simulink model "extforce_free_orbit_box"  (R2019b)
settings: Solver=ode45  StartTime=0.0  StopTime=20000.0  MaxStep=0.01  RelTol=1e-8
settings Model: Creator=Hector  LastModifiedBy=Hector

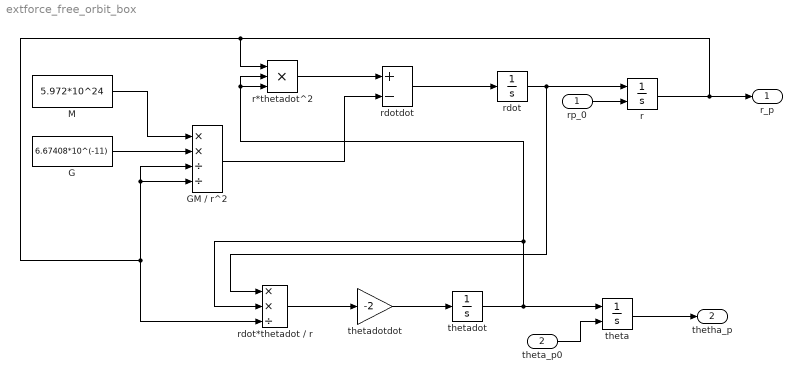
== system extforce_free_orbit_box ==
  rp_0 : Inport
  theta_p0 : Inport  Port=2
  G : Constant  Value=6.67408*10^(-11)
  GM / r^2 : Product  Inputs=**//
  M : Constant  Value=5.972*10^24
  r : Integrator  InitialConditionSource=external  InitialCondition=6.7871*10^6
  r*thetadot^2 : Product  Inputs=3
  rdot : Integrator
  rdot*thetadot / r : Product  Inputs=**/
  rdotdot : Sum  Inputs=+-
  theta : Integrator  InitialConditionSource=external  InitialCondition=pi/4
  thetadot : Integrator  InitialCondition=0.001129091743116
  thetadotdot : Gain  Gain=-2
  r_p : Outport
  thetha_p : Outport  Port=2
  wires:
  M/1 -> GM / r^2/1
  G/1 -> GM / r^2/2
  r*thetadot^2/1 -> rdotdot/1
  GM / r^2/1 -> rdotdot/2
  rdotdot/1 -> rdot/1
  thetadot/1 -> r*thetadot^2/2, r*thetadot^2/3, rdot*thetadot / r/2, theta/1
  rdot*thetadot / r/1 -> thetadotdot/1
  rdot/1 -> rdot*thetadot / r/1, r/1
  thetadotdot/1 -> thetadot/1
  r/1 -> rdot*thetadot / r/3, GM / r^2/3, GM / r^2/4, r*thetadot^2/1, r_p/1
  theta/1 -> thetha_p/1
  rp_0/1 -> r/2
  theta_p0/1 -> theta/2
